simulink model "GS_LQI_problem"  (R2023b)
settings: Solver=VariableStepAuto  StartTime=0.0  StopTime=10.0  RelTol=1e-3
settings Model: Creator=giova  LastModifiedBy=miche

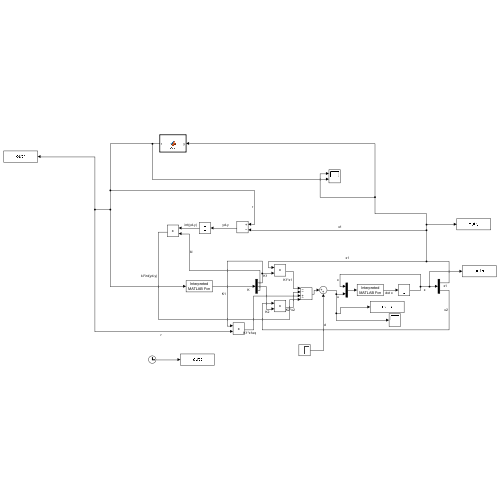
[thumbnail: Simulink's stored preview of the top-level diagram]
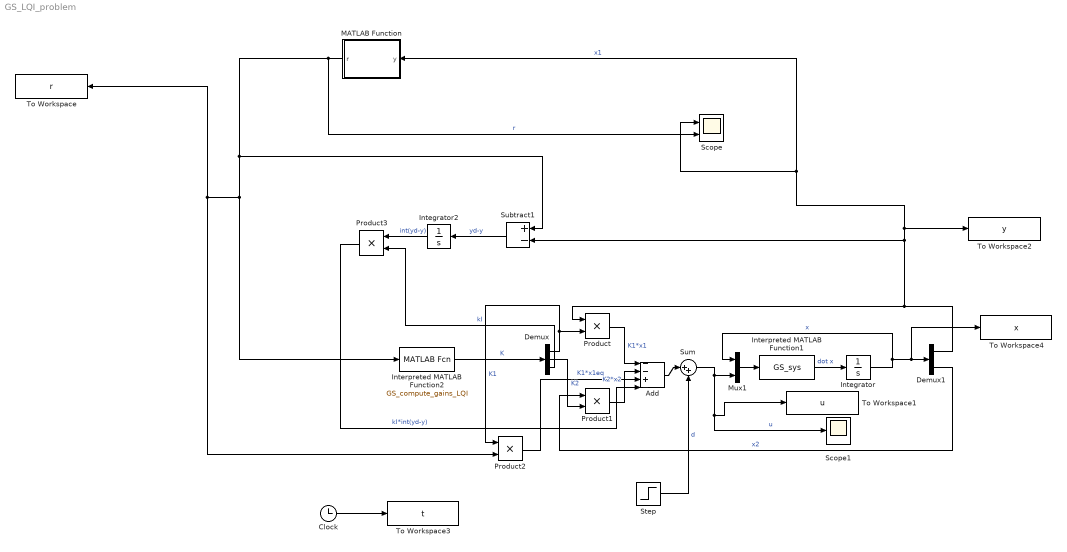
== system GS_LQI_problem ==
  Add : Sum  Inputs=--+-
  Clock : Clock
  Demux : Demux  Outputs=3
  Demux1 : Demux  Outputs=2
  Integrator : Integrator
  Integrator2 : Integrator
  Interpreted MATLAB Function1 : MATLABFcn  MATLABFcn=GS_sys  OutputDimensions=2
  Interpreted MATLAB Function2 : MATLABFcn  MATLABFcn=GS_compute_gains_LQI  OutputDimensions=3
  MATLAB Function : MATLAB Function  TreatAsAtomicUnit=on
  Mux1 : Mux  Inputs=2
  Product{,1..3} (4 alike) : Product
  Scope : Scope  NumInputPorts=2
  Scope1 : Scope
  Step : Step  Time=5  After=350  SampleTime=0
  Subtract1 : Sum  Inputs=+-
  Sum : Sum  Inputs=|++
  To Workspace : ToWorkspace  VariableName=r  SampleTime=-1
  To Workspace1 : ToWorkspace  VariableName=u  SampleTime=-1
  To Workspace2 : ToWorkspace  VariableName=y  SampleTime=-1
  To Workspace3 : ToWorkspace  VariableName=t  SampleTime=-1
  To Workspace4 : ToWorkspace  VariableName=x  SampleTime=-1
  wires:
  Interpreted MATLAB Function1/1 -> Integrator/1  "dot x"
  Step/1 -> Sum/2  "d"
  Product2/1 -> Add/3  "K1*x1eq"
  Subtract1/1 -> Integrator2/1  "yd-y"
  Demux1/2 -> Product1/1  "x2"
  Demux1/1 -> Product/1, MATLAB Function/1(y), Scope/1, To Workspace2/1, Subtract1/2  "x1"
  Add/1 -> Sum/1
  Mux1/1 -> Interpreted MATLAB Function1/1
  Product3/1 -> Add/4  "kI*int(yd-y)"
  Integrator2/1 -> Product3/1  "int(yd-y)"
  Demux/2 -> Product1/2  "K2"
  Interpreted MATLAB Function2/1 -> Demux/1  "K"
  MATLAB Function/1(r) -> Scope/2, Product2/2, To Workspace/1, Interpreted MATLAB Function2/1, Subtract1/1  "r"
  Product/1 -> Add/1  "K1*x1"
  Demux/3 -> Product3/2  "kI"
  Integrator/1 -> To Workspace4/1, Demux1/1, Mux1/1  "x"
  Demux/1 -> Product2/1, Product/2  "K1"
  Clock/1 -> To Workspace3/1
  Sum/1 -> Mux1/2, To Workspace1/1, Scope1/1  "u"
  Product1/1 -> Add/2  "K2*x2"

== matlab function GS_LQI_problem/MATLAB Function ==
  data: y input; r output
function r = fcn(y)
    if(y==0)
        r=pi;
    else
        r=fix(y/(2*pi))*2*pi + pi*sign(y);
    end
end
